simulink model "ackerman_ROS_neural_controller"  (R2023b)
settings: Solver=FixedStepDiscrete  StartTime=0.0  StopTime=20  FixedStep=0.1  RelTol=1e-3
undefined symbols (not defined in the file or in its folder): Angular, Linear
libraries: neural x61, robotlib x15, robotcorelib x1
(part 3 of 3)

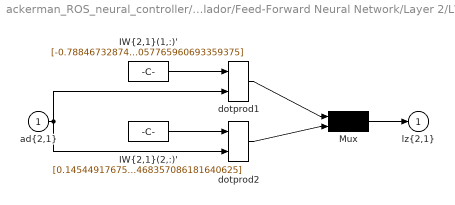
== system ackerman_ROS_neural_controller/Controlador/Feed-Forward Neural Network/Layer 2/LW{2,1} ==
  "ad{2,1}" : Inport  PortDimensions=55
      mask Display: e = 0.06;c1 = [120 230 180]/255;c2 = ([120 230 180]+0)/(256+128);c3 = ([120 230 180]+128)/(256+128);patch([0 1 1 0],[0 0 1 1],c1);patch([0 1 1 1-e 1-e 0+e],[0 0 1 1-e 0+e 0+e],c2);patch([0 0 1 1-e 0+e 0+e],[0 1 1 1-e 1-e 0+e],c3);plot([0 1 1 0 0],[0 0 1 1 0]);
  "IW{2,1}(1,:)'" : Constant  Value=[-0.78846732874251335143611640887684188783168792724609375;1.8691073983835073679671268109814263880252838134765625;-1.054597751008004902217862763791345059871673583984375;0.83328992903374266010274595828377641737461090087890625;0.430278758730233745755100471797049976885318756103515625;1.2514847056409668102361365527031011879444122314453125;1.24987536579162483718619114370085299015045166015625;1.4580140848525982022465541376732289791107177734375;-1.291630812550348395006949431262910366058349609375;-0.7108099844022159885525979916565120220184326171875;-0.362778693733005919153100649054977111518383026123046875;-0.58121311187843804901831390452571213245391845703125;1.0118358400578613132125838092179037630558013916015625;-2.217770394869860606235079103498719632625579833984375;-1.6634221098131265481612217627116478979587554931640625;-1.5119149791612878086510818320675753057003021240234375;0.55848817890764113069934637678670696914196014404296875;0.207509560696907902066499218562967143952846527099609375;3.53587165791001556414130391203798353672027587890625;-0.85143721780173386992629502856289036571979522705078125;-0.630050438856013528265975764952600002288818359375;1.10864992313193067019483351032249629497528076171875;1.21924251577572473337340852594934403896331787109375;1.1708998236688545890871182564296759665012359619140625;0.5319693222242556362999721386586315929889678955078125;2.3404277299213216423368066898547112941741943359375;1.3153000806466292882390689555904828011989593505859375;-0.2318105505096202112458314559262362308800220489501953125;-1.8388804996603338448579734176746569573879241943359375;-1.61085978217581793359158837120048701763153076171875;0.5686703429631621009576747383107431232929229736328125;1.4867363420598656009730120786116458475589752197265625;-1.536349307105904671288953977636992931365966796875;-1.492010078414608642560779117047786712646484375;1.477475905074709938702426370582543313503265380859375;0.818303793350279473628461346379481256008148193359375;1.008521170471887717923209493164904415607452392578125;0.7215425460949915770214602162013761699199676513671875;-0.95785326859383690401017474869149737060070037841796875;-1.505958079256698223247212808928452432155609130859375;-1.34955975313096931955669788294471800327301025390625;-0.47778192278437658924161723916768096387386322021484375;-2.67380015214178801130628926330246031284332275390625;-0.134018909238493744151554665222647599875926971435546875;-2.29042260255578522532005081302486360073089599609375;-0.92448969355089538613157174040679819881916046142578125;-1.5621878454640591993296538930735550820827484130859375;0.5795268702875231436877356827608309686183929443359375;-0.6310960677225969650550041478709317743778228759765625;0.0871809844683806012266558127521420828998088836669921875;-1.69550833967105152311205529258586466312408447265625;0.3036517789830792679595106164924800395965576171875;-0.117837271324522152582403577980585396289825439453125;1.2525125459518584580820288465474732220172882080078125;-0.1396963359400368032137151885763159953057765960693359375]
      mask Display: e = 0.06;c1 = [120 150 230]/255;c2 = ([120 150 230]+0)/383;c3 = ([120 150 230]+128)/383;patch([0 1 1 0],[0 0 1 1],c1);patch([0 1 1 1-e 1-e 0+e],[0 0 1 1-e 0+e 0+e],c2);patch([0 0 1 1-e 0+e 0+e],[0 1 1 1-e 1-e 0+e],c3);plot([0 1 1 0 0],[0 0 1 1 0]);disp('weights');
  "IW{2,1}(2,:)'" : Constant  Value=[0.14544917675115265343066539571736939251422882080078125;0.316821076978230420362336872130981646478176116943359375;-0.378574076100946455003537494121701456606388092041015625;-0.0204587120000312150391863497134181670844554901123046875;0.625786585156384855821443125023506581783294677734375;0.6714967906168387568044408908463083207607269287109375;-0.27018335172530871801654939190484583377838134765625;0.8413491475219496695814314080053009092807769775390625;1.0485464784718099284788195291184820234775543212890625;0.0182542404893475014582282511810262803919613361358642578125;0.9284305817833897744861815226613543927669525146484375;-0.5645876146983119792110983325983397662639617919921875;0.16042019508611493616712095899856649339199066162109375;0.85139096859865792676913542891270481050014495849609375;-0.3309262502250247539592464818269945681095123291015625;-0.1061610777999584254160936325206421315670013427734375;0.375174846765524649949696822659461759030818939208984375;0.0265377576715836449583463263479643501341342926025390625;0.109546557540195210744826681548147462308406829833984375;0.08798409881725921533046630429453216493129730224609375;-0.8183699597635640810011636858689598739147186279296875;-0.55263537384756900028293102877796627581119537353515625;-0.133962660880776684990678404574282467365264892578125;-0.23811817946833147008334208294400013983249664306640625;0.99355535902571123774151828911271877586841583251953125;-0.0829149883129794151859215389777091331779956817626953125;-0.0826747734261817079914891337466542609035968780517578125;0.8378716644694395032644251841702498495578765869140625;0.14384525431915096138624221566715277731418609619140625;0.7289259815840527512165181178716011345386505126953125;0.21377103995719848317236255752504803240299224853515625;0.1933583239805957421086901604212471283972263336181640625;0.234424213760843380693899007383151911199092864990234375;0.09034397614492929717844305059770704247057437896728515625;-0.34197661012264635171931104196119122207164764404296875;-0.40847865386311543733910411901888437569141387939453125;0.302963061133577848949016697588376700878143310546875;-0.5181686606488649093904541587107814848423004150390625;-0.7190868338323308517345822110655717551708221435546875;-0.453215365618822918492014650837518274784088134765625;-0.428815371161506864172707764737424440681934356689453125;-0.50333346104687393118837235306273214519023895263671875;0.1965635546835204916504835637169890105724334716796875;0.26679747073666160162019878043793141841888427734375;0.0213368290357197655515708589746282086707651615142822265625;0.490029304191835157755718910266296006739139556884765625;-0.9957349315888255336659540262189693748950958251953125;-0.229310188867238640142431904678232967853546142578125;1.1936314866180544047580269761965610086917877197265625;-0.56118382975087810482506256448687054216861724853515625;-0.0630123421789567095263606688604340888559818267822265625;-0.06552508964497176513486209614711697213351726531982421875;0.53661024344239172112480673604295589029788970947265625;-0.34435362767606758627181307019782252609729766845703125;-0.0308784756067243849886327922149575897492468357086181640625]
      mask Display: e = 0.06;c1 = [120 150 230]/255;c2 = ([120 150 230]+0)/383;c3 = ([120 150 230]+128)/383;patch([0 1 1 0],[0 0 1 1],c1);patch([0 1 1 1-e 1-e 0+e],[0 0 1 1-e 0+e 0+e],c2);patch([0 0 1 1-e 0+e 0+e],[0 1 1 1-e 1-e 0+e],c3);plot([0 1 1 0 0],[0 0 1 1 0]);disp('weights');
  Mux : Mux  Inputs=2
      mask Display: e = 0.06;c1 = [120 150 230]/255;c2 = ([120 150 230]+0)/383;c3 = ([120 150 230]+128)/383;patch([0 1 1 0],[0 0 1 1],c1);patch([0 1 1 1-e 1-e 0+e],[0 0 1 1-e 0+e 0+e],c2);patch([0 0 1 1-e 0+e 0+e],[0 1 1 1-e 1-e 0+e],c3);plot([0 1 1 0 0],[0 0 1 1 0]);disp('Mux');
  dotprod1 : neural/Weight Functions/dotprod
  dotprod2 : neural/Weight Functions/dotprod
  "lz{2,1}" : Outport
      mask Display: e = 0.06;c1 = [120 230 180]/255;c2 = ([120 230 180]+0)/(256+128);c3 = ([120 230 180]+128)/(256+128);patch([0 1 1 0],[0 0 1 1],c1);patch([0 1 1 1-e 1-e 0+e],[0 0 1 1-e 0+e 0+e],c2);patch([0 0 1 1-e 0+e 0+e],[0 1 1 1-e 1-e 0+e],c3);plot([0 1 1 0 0],[0 0 1 1 0]);
  wires:
  "IW{2,1}(1,:)'"/1 -> dotprod1/1
  "ad{2,1}"/1 -> dotprod1/2, dotprod2/2
  dotprod1/1 -> Mux/1
  "IW{2,1}(2,:)'"/1 -> dotprod2/1
  dotprod2/1 -> Mux/2
  Mux/1 -> "lz{2,1}"/1

== matlab function ackerman_ROS_neural_controller/ROS Robot/Conversion_diff_ackerman ==
  data: steering_wheel_angle input; V output; linear_vel_ackerman_kmh input; W output
function [V,W] = fcn(steering_wheel_angle, linear_vel_ackerman_kmh)

    %Aproximacion de angulo volante y velocidad linal a vel_linar y angular.
    % *************************************
    
    min_turning_radius_vehicle = 2;  % radio de giro del vehiculo. Radio minimo en el que gira 180 grados. 
    max_turning_radius_vehicle = 34; % radio de giro del vehiculo. Radio máximo con el volante girado 1º
    max_steering_wheel_angle = 90;  % angulo máximo de volante permitido (grados).
    max_vehicle_linear_speed = 30;  % velocidad máxima de vehiculo (km/h).
    
    
    % Filtrado des los valores máximos
    
    if steering_wheel_angle > max_steering_wheel_angle
        steering_wheel_angle = max_steering_wheel_angle;  
    end
    
    if steering_wheel_angle < (-1*max_steering_wheel_angle)
        steering_wheel_angle = max_steering_wheel_angle;  
    end
    
    if linear_vel_ackerman_kmh > max_vehicle_linear_speed
        linear_vel_ackerman_kmh = max_vehicle_linear_speed;
    end
    
    
    %Conversion a m/s
    linear_vel_ackerman_ms = linear_vel_ackerman_kmh/3.6; %(m/s)
    
    %Conversion a linear and angular velocity for the simulator.
    % v=rω --> ω = v/r
    
    % max_steering_wheel_angle -- > min_turning_radius_vehicle
    % steering_wheel_angle = 0 --> angular_vel_vehicle = 0;
    
    turning_radius = (max_turning_radius_vehicle-((max_turning_radius_vehicle-min_turning_radius_vehicle)/max_steering_wheel_angle)*abs(steering_wheel_angle));
    
    if steering_wheel_angle > 0
            turning_radius = turning_radius;
    elseif steering_wheel_angle < 0
            turning_radius = -1*turning_radius;
    end
    
    if abs(steering_wheel_angle) < 0.01
        angular_vel_vehicle = 0;
    else
        angular_vel_vehicle = linear_vel_ackerman_ms / turning_radius;
    end
    
    %Sin velocidad linear, tampoco debe girar
    
    if linear_vel_ackerman_ms == 0
        angular_vel_vehicle = 0;
    end
    
    
    %Rellenamos los campos del mensaje V y W
    V= linear_vel_ackerman_ms;

    W=angular_vel_vehicle;
    
    
    %********************************************************

== matlab function ackerman_ROS_neural_controller/ROS Robot/MATLAB Function ==
  data: u input; y output
function y = fcn(u)
u(isinf(u))=5.0;
y = u;

== matlab function ackerman_ROS_neural_controller/Condicion de Parada ==
  data: flag_parada output; raw_speed input; filter_speed output; sens input
function [flag_parada, filter_speed] = condicion_parada(raw_speed, sens)

% Condicion de parada:
% - debeis decidir cuando se finaliza la maniobra de aparcamiento en base
%  a la información disponible:
%      - velocidad_lineal
%      - ángulo de volante      
%      - sensores
% Una vez que decidais cual es el criterio de parada debeis:
%   - Parar el vehículo con v_lineal = 0.
%   - Activar el flag_parada a 1 para indicar que ha finalizado la maniobra.

if ~ismember(0, sens) && sens(4) <= 0.5 && sens(5) <= 0.5 % Ejemplo de condición de parada

    %Es necesario parar el vehículo con v_lineal = 0 y activar el
    %flag_parada a 1 para indicar que ha finalizado la maniobra.
    filter_speed = 0.0;
    flag_parada=1;

elseif ismember(0, sens)
    filter_speed = 0.0;
    flag_parada=0;

else
    filter_speed = raw_speed;
    flag_parada=0;
end

== matlab function ackerman_ROS_neural_controller/Evaluacion_maniobra/Evaluacion_fin_maniobra ==
  data: clock input; flag_parada input; x input; y input; theta input; stop_flag output
function stop_flag = evaluacion_maniobra(clock, flag_parada, x, y, theta)

if flag_parada == 1

    parking_time = clock
    parking_position_x = x
    parking_position_y = y
    parking_position_theta = theta
    stop_flag = 1;
else
    stop_flag = 0;

end
